simulink model "PrimerEjercicio"  (R2018a)
settings: Solver=VariableStepAuto  StartTime=0.0  StopTime=100  RelTol=1e-3
settings Model: Creator=ESTUDIANTE  LastModifiedBy=ESTUDIANTE

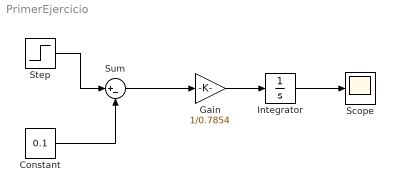
== system PrimerEjercicio ==
  Constant : Constant  Value=0.1
  Gain : Gain  Gain=1/0.7854
  Integrator : Integrator  InitialCondition=1
  Scope : Scope
  Step : Step  Before=0.1  After=0.11  SampleTime=0
  Sum : Sum  Inputs=|+-
  wires:
  Constant/1 -> Sum/2
  Step/1 -> Sum/1
  Sum/1 -> Gain/1
  Gain/1 -> Integrator/1
  Integrator/1 -> Scope/1
